simulink model "OpdrachtDeel2SimulinkSine"  (R2016b)
settings: Solver=FixedStepAuto  StartTime=0.0  StopTime=100  FixedStep=0.001  RelTol=1e-3
settings Model: Creator=User  LastModifiedBy=User

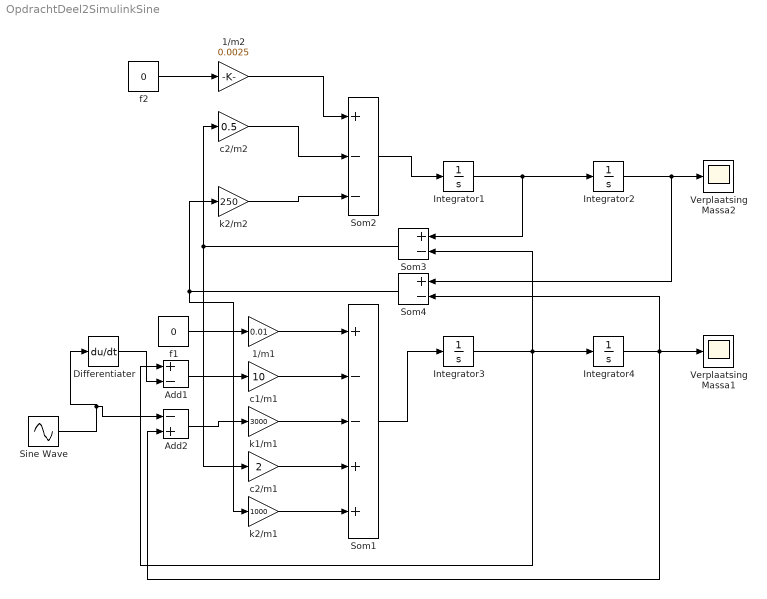
== system OpdrachtDeel2SimulinkSine ==
  1/m1 : Gain  Gain=0.01
  1/m2 : Gain  Gain=0.0025
  Add1 : Sum  Inputs=+-
  Add2 : Sum  Inputs=-+
  Differentiater : Derivative
  Integrator{1..4} (4 alike) : Integrator
  Sine Wave : Sin  Amplitude=0.02  Frequency=5  SampleTime=0
  Som1 : Sum  Inputs=+--++
  Som2 : Sum  Inputs=+--
  Som3 : Sum  Inputs=+-
  Som4 : Sum  Inputs=+-
  Verplaatsing Massa1 : Scope
  Verplaatsing Massa2 : Scope
  c1/m1 : Gain  Gain=10
  c2/m1 : Gain  Gain=2
  c2/m2 : Gain  Gain=0.5
  f1 : Constant  Value=0
  f2 : Constant  Value=0
  k1/m1 : Gain  Gain=3000
  k2/m1 : Gain  Gain=1000
  k2/m2 : Gain  Gain=250
  wires:
  Integrator1/1 -> Som3/1, Integrator2/1
  Integrator2/1 -> Som4/1, Verplaatsing Massa2/1
  Som2/1 -> Integrator1/1
  c2/m2/1 -> Som2/2
  k2/m2/1 -> Som2/3
  1/m2/1 -> Som2/1
  f2/1 -> 1/m2/1
  Som3/1 -> c2/m1/1, c2/m2/1
  Integrator4/1 -> Add2/2, Som4/2, Verplaatsing Massa1/1
  Som1/1 -> Integrator3/1
  Integrator3/1 -> Add1/1, Som3/2, Integrator4/1
  k2/m1/1 -> Som1/5
  c2/m1/1 -> Som1/4
  k1/m1/1 -> Som1/3
  c1/m1/1 -> Som1/2
  1/m1/1 -> Som1/1
  f1/1 -> 1/m1/1
  Add1/1 -> c1/m1/1
  Add2/1 -> k1/m1/1
  Differentiater/1 -> Add1/2
  Som4/1 -> k2/m1/1, k2/m2/1
  Sine Wave/1 -> Differentiater/1, Add2/1
